simulink model "EsSinc"  (R2017a)
settings: Solver=FixedStepDiscrete  StartTime=0.0  StopTime=inf  RelTol=1e-3
settings Model: Creator=Fabio  LastModifiedBy=Fabio
settings DataIOCC: LimitDataPoints=on  SaveOutput=off  SaveTime=off
settings OptimizationCC: BooleanDataType=off  DefaultParameterBehavior=Inlined  LocalBlockOutputs=off  LifeSpan=inf
settings DebuggingCC: AlgebraicLoopMsg=error  SingleTaskRateTransMsg=error  AllowSymbolicDim=off  SFUnexpectedBacktrackingDiag=warning  SFNoUnconditionalDefaultTransitionDiag=warning  SFExecutionAtInitializationDiag=none
settings GRTTargetCC: TargetLangStandard=C89/C90 (ANSI)  GeneratePreprocessorConditionals=Disable all
settings ConfigComp: CovMetricSettings=dw  CovHtmlReporting=on  CovSaveCumulativeToWorkspaceVar=on  CovSaveSingleToWorkspaceVar=on  CovExternalEMLEnable=off  CovSFcnEnable=off

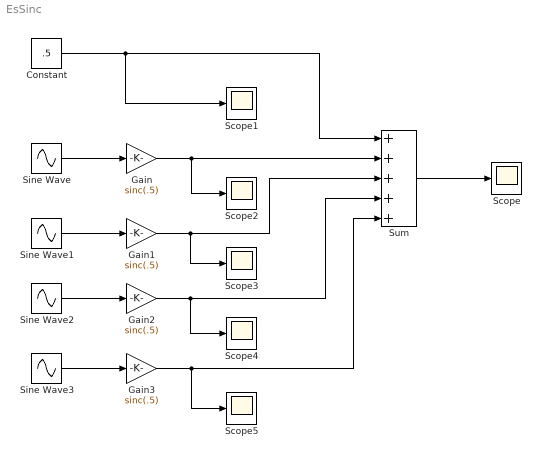
== system EsSinc ==
  Constant : Constant  Value=.5  SampleTime=0.001
  Gain{,1..3} (4 alike) : Gain  Gain=sinc(.5)
  Scope{,1..5} (6 alike) : Scope
  Sine Wave{,1..3} (4 alike) : Sin  Frequency=2*pi  Phase=pi/2  SampleTime=0.001
  Sum : Sum  Inputs=+++++
  wires:
  Constant/1 -> Scope1/1, Sum/1
  Sum/1 -> Scope/1
  Sine Wave/1 -> Gain/1
  Sine Wave1/1 -> Gain1/1
  Sine Wave2/1 -> Gain2/1
  Sine Wave3/1 -> Gain3/1
  Gain/1 -> Scope2/1, Sum/2
  Gain1/1 -> Scope3/1, Sum/3
  Gain2/1 -> Scope4/1, Sum/4
  Gain3/1 -> Scope5/1, Sum/5
